simulink model "adapHCS_model"  (R2022b)
settings: Solver=VariableStepAuto  StartTime=0.0  StopTime=t_sample*n_sample  MaxStep=15  MinStep=10  RelTol=1e-3
values from neighbouring files (symbols this model uses):
  air_den = 1.225    [wind_turbine_parameters.m]
  l1 = 56    [wind_turbine_parameters.m]
  t_sample = 10*60    (= 600)    [wind_turbine_parameters.m]
undefined symbols (not defined in the file or in its folder): pitch_deg
libraries: simulink x1
settings Model: PacingRate=1000  Creator=luan  LastModifiedBy=marina
settings SolverCC: ZeroCrossAlgorithm=Adaptive
settings DebuggingCC: IgnoredZcDiagnostic=none
settings ConfigComp: CovScope=ReferencedModels

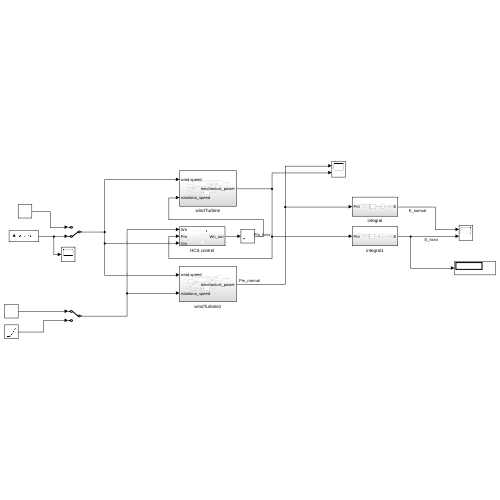
[thumbnail: Simulink's stored preview of the top-level diagram]
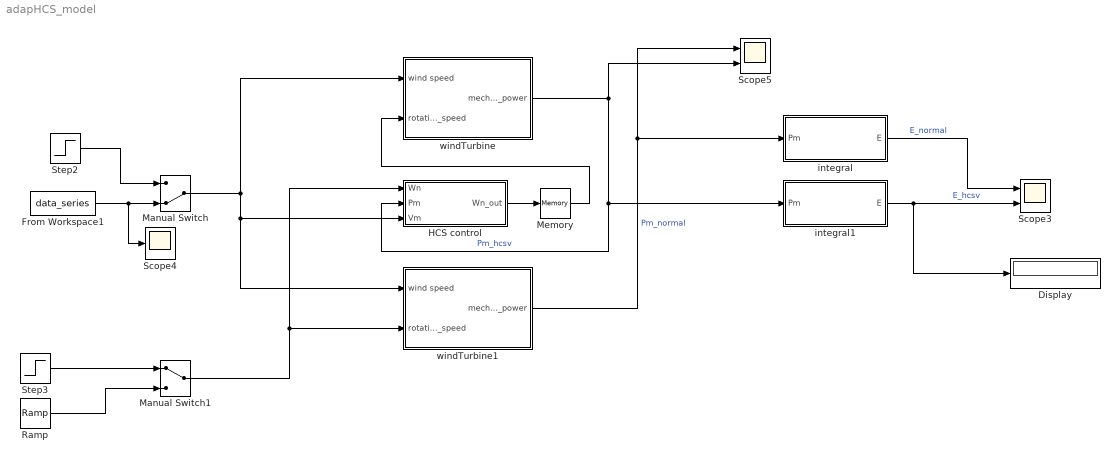
== system adapHCS_model ==
  Display : Display
  From Workspace1 : FromWorkspace  VariableName=data_series  SampleTime=t_sample  OutputAfterFinalValue=Setting to zero
  HCS control : Subsystem
  Manual Switch : ManualSwitch  CurrentSetting=0
  Manual Switch1 : ManualSwitch
  Memory : Memory
  Ramp : simulink/Sources/Ramp  slope=0.000007  start=0  InitialOutput=0.0001
  Scope3 : Scope  NumInputPorts=2
  Scope4 : Scope
  Scope5 : Scope  NumInputPorts=2
  Step2 : Step  Time=0  After=10  SampleTime=0
  Step3 : Step  Time=0  SampleTime=0
  integral : Subsystem
  integral1 : Subsystem
  windTurbine : Subsystem
  windTurbine1 : Subsystem
  wires:
  windTurbine1/1(mechanical_power) -> Scope5/1, integral/1(Pm)  "Pm_normal"
  windTurbine/1(mechanical_power) -> Scope5/2, HCS control/2(Pm), integral1/1(Pm)  "Pm_hcsv"
  Step2/1 -> Manual Switch/1
  From Workspace1/1 -> Scope4/1, Manual Switch/2
  Step3/1 -> Manual Switch1/1
  Ramp/1 -> Manual Switch1/2
  HCS control/1(Wn_out) -> Memory/1
  integral1/1(E) -> Display/1, Scope3/2  "E_hcsv"
  Memory/1 -> windTurbine/2(rotationa_speed)
  integral/1(E) -> Scope3/1  "E_normal"
  Manual Switch1/1 -> HCS control/1(Wn), windTurbine1/2(rotationa_speed)
  Manual Switch/1 -> windTurbine/1(wind speed), windTurbine1/1(wind speed), HCS control/3(Vm)

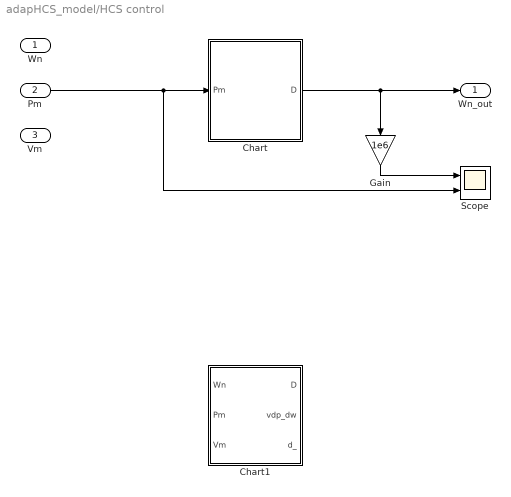
== system adapHCS_model/HCS control ==
  Wn : Inport
  Pm : Inport  Port=2
  Vm : Inport  Port=3
  Chart : Stateflow chart  TreatAsAtomicUnit=on
  Chart1 : Stateflow chart  TreatAsAtomicUnit=on
  Gain : Gain  Gain=1e6
  Scope : Scope  NumInputPorts=2
  Wn_out : Outport
  wires:
  Chart/1(D) -> Gain/1, Wn_out/1
  Pm/1 -> Scope/2, Chart/1(Pm)
  Gain/1 -> Scope/1

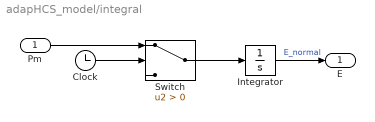
== system adapHCS_model/integral ==
  Pm : Inport
  Clock : Clock
  Integrator : Integrator
  Switch : Switch  Criteria=u2 > Threshold  SaturateOnIntegerOverflow=off  InputSameDT=off
  E : Outport
  wires:
  Switch/1 -> Integrator/1
  Clock/1 -> Switch/2
  Pm/1 -> Switch/1
  Integrator/1 -> E/1  "E_normal"

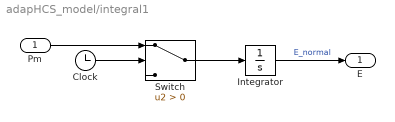
== system adapHCS_model/integral1 ==
  Pm : Inport
  Clock : Clock
  Integrator : Integrator
  Switch : Switch  Criteria=u2 > Threshold  SaturateOnIntegerOverflow=off  InputSameDT=off
  E : Outport
  wires:
  Integrator/1 -> E/1  "E_normal"
  Pm/1 -> Switch/1
  Clock/1 -> Switch/2
  Switch/1 -> Integrator/1

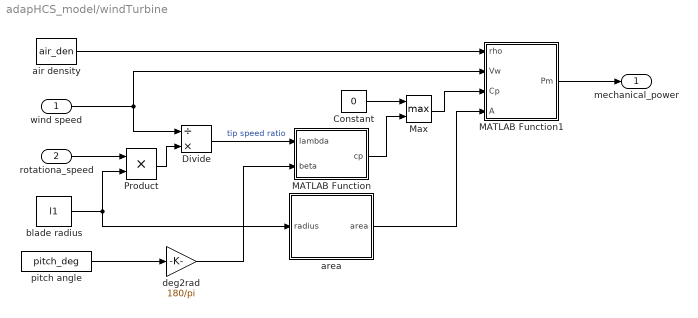
== system adapHCS_model/windTurbine ==
  wind speed : Inport
  rotationa_speed : Inport  Port=2
  Constant : Constant  Value=0
  Divide : Product  Inputs=/*
  MATLAB Function : MATLAB Function  TreatAsAtomicUnit=on
  MATLAB Function1 : MATLAB Function  TreatAsAtomicUnit=on
  Max : MinMax  Function=max  Inputs=2
  Product : Product
  air density : Constant  Value=air_den
  area : Subsystem
  blade radius : Constant  Value=l1
  deg2rad : Gain  Gain=180/pi
  pitch angle : Constant  Value=pitch_deg
  mechanical_power : Outport
  wires:
  Product/1 -> Divide/2
  wind speed/1 -> Divide/1, MATLAB Function1/2(Vw)
  Divide/1 -> MATLAB Function/1(lambda)  "tip speed ratio"
  MATLAB Function1/1(Pm) -> mechanical_power/1
  rotationa_speed/1 -> Product/1
  air density/1 -> MATLAB Function1/1(rho)
  area/1(area) -> MATLAB Function1/4(A)
  blade radius/1 -> Product/2, area/1(radius)
  deg2rad/1 -> MATLAB Function/2(beta)
  Max/1 -> MATLAB Function1/3(Cp)
  MATLAB Function/1(cp) -> Max/2
  Constant/1 -> Max/1
  pitch angle/1 -> deg2rad/1

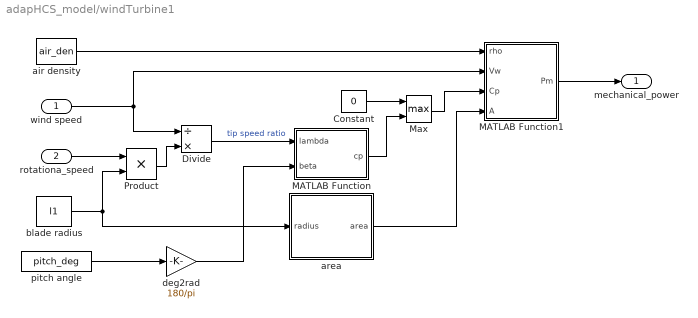
== system adapHCS_model/windTurbine1 ==
  wind speed : Inport
  rotationa_speed : Inport  Port=2
  Constant : Constant  Value=0
  Divide : Product  Inputs=/*
  MATLAB Function : MATLAB Function  TreatAsAtomicUnit=on
  MATLAB Function1 : MATLAB Function  TreatAsAtomicUnit=on
  Max : MinMax  Function=max  Inputs=2
  Product : Product
  air density : Constant  Value=air_den
  area : Subsystem
  blade radius : Constant  Value=l1
  deg2rad : Gain  Gain=180/pi
  pitch angle : Constant  Value=pitch_deg
  mechanical_power : Outport
  wires:
  Product/1 -> Divide/2
  wind speed/1 -> Divide/1, MATLAB Function1/2(Vw)
  Divide/1 -> MATLAB Function/1(lambda)  "tip speed ratio"
  MATLAB Function1/1(Pm) -> mechanical_power/1
  rotationa_speed/1 -> Product/1
  air density/1 -> MATLAB Function1/1(rho)
  area/1(area) -> MATLAB Function1/4(A)
  blade radius/1 -> Product/2, area/1(radius)
  deg2rad/1 -> MATLAB Function/2(beta)
  Max/1 -> MATLAB Function1/3(Cp)
  MATLAB Function/1(cp) -> Max/2
  Constant/1 -> Max/1
  pitch angle/1 -> deg2rad/1

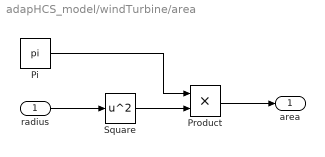
== system adapHCS_model/windTurbine/area ==
  radius : Inport
  Pi : Constant  Value=pi  OutDataTypeStr=Inherit: Inherit via back propagation
  Product : Product
  Square : Math  Operator=square
  area : Outport
  wires:
  radius/1 -> Square/1
  Square/1 -> Product/2
  Pi/1 -> Product/1
  Product/1 -> area/1

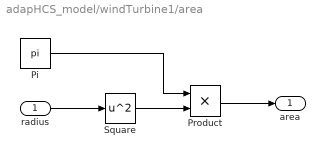
== system adapHCS_model/windTurbine1/area ==
  radius : Inport
  Pi : Constant  Value=pi  OutDataTypeStr=Inherit: Inherit via back propagation
  Product : Product
  Square : Math  Operator=square
  area : Outport
  wires:
  radius/1 -> Square/1
  Square/1 -> Product/2
  Pi/1 -> Product/1
  Product/1 -> area/1

== stateflow chart adapHCS_model/HCS control/Chart ==
  state init_
    entry:
    D = 1;
    pt_1 = Pm;
    direction = 1;
  state perturb_
    entry:
    D = D + d_;
    D = max(D, 0);
    pt_1 = Pm;
  state measure
    entry:
    dp = Pm - pt_1;
  state keep_direction
    entry:
    direction = direction;
  state update
    entry:
    d_ = direction * Gamma * abs(dp);
  state change_direction
    entry:
    direction = -1* direction;
  state perturb
    entry:
    d_ = randn(1)/500;
    direction = d_/abs(d_);
  (junction 73) -> (junction 74)
  (default) -> init_
  (junction 74) -> measure
  (junction 77) -> (junction 73)
  update -> perturb_
  init_ -> measure
  measure -> keep_direction [order 2] : [dp > Tr]
  keep_direction -> update
  perturb_ -> (junction 77) : [after(delay,sec)]
  (junction 99) -> update
  measure -> perturb [order 3]
  measure -> (junction 95) [order 1] : [dp < -Tr]
  (junction 121) -> perturb_
  (junction 95) -> change_direction
  change_direction -> (junction 99)
  perturb -> (junction 121)
  data: Pm input; D output; delay constant double =30; pt_1 local =1000; dp local; Gamma constant double =1e-7; d_ local; direction local; Tr constant double

== matlab function adapHCS_model/windTurbine/MATLAB Function ==
  data: lambda input; cp output; beta input
function cp = fcn(lambda, beta)

k = load('coefficients.mat');
lambda_i =  1/(1/(lambda + 0.08*beta) - 0.035/(1+beta*beta*beta));

% Debug
% lambda_i
% k.k1 *(k.k2/lambda_i - k.k3*beta - k.k4*power(beta, k.k5) -k.k6)*exp(-k.k7/lambda_i)

cp = k.k1 *(k.k2/lambda_i - k.k3*beta - k.k4*power(beta, k.k5) -k.k6)*exp(-k.k7/lambda_i);

== matlab function adapHCS_model/windTurbine1/MATLAB Function ==
  data: lambda input; cp output; beta input
function cp = fcn(lambda, beta)

k = load('coefficients.mat');
lambda_i =  1/(1/(lambda + 0.08*beta) - 0.035/(1+beta*beta*beta));

% Debug
% lambda_i
% k.k1 *(k.k2/lambda_i - k.k3*beta - k.k4*power(beta, k.k5) -k.k6)*exp(-k.k7/lambda_i)

cp = k.k1 *(k.k2/lambda_i - k.k3*beta - k.k4*power(beta, k.k5) -k.k6)*exp(-k.k7/lambda_i);

== matlab function adapHCS_model/windTurbine1/MATLAB Function1 ==
  data: rho input; Vw input; Pm output; Cp input; A input
function Pm = fcn(rho, Vw, Cp, A)

Pm = 0.5* Cp* rho* A* power(Vw, 3);

== matlab function adapHCS_model/windTurbine/MATLAB Function1 ==
  data: rho input; Vw input; Pm output; Cp input; A input
function Pm = fcn(rho, Vw, Cp, A)

Pm = 0.5* Cp* rho* A* power(Vw, 3);

== stateflow chart adapHCS_model/HCS control/Chart1 ==
  state stationary
    entry:
    D = Wn;
  state measure
    entry:
    dp = Pm - pt_1;
    dw = D-wn_1;
    pt_1 = Pm;
    wn_1 = D;
    vdp_dw =  Vm*dp/dw;
  state decrease
    entry:
  state decrease_a_lot
    entry:
    d_ = - d_lot;
  state init_
    entry:
    D = Wn;
    pt_1 = 0;
    wn_1 = 0;
    vdp_dw_1 = 0;
  state decrease_a_bit
    entry:
    d_ = - d_bit;
  state perturb_
    entry:
    D = D + d_;
    vdp_dw_1 = vdp_dw;
  state increase_a_bit
    entry:
    d_ = d_bit;
  state increase
    entry:
  state increase_a_lot
    entry:
    d_ = d_lot;
  measure -> stationary [order 3] : [dp==0]
  stationary -> measure : [after(delay,sec)]
  (junction 73) -> (junction 74)
  (junction 74) -> measure
  (junction 77) -> (junction 73)
  (default) -> init_
  decrease_a_lot -> (junction 66)
  measure -> decrease [order 2] : [dp < 0]
  decrease -> decrease_a_lot [order 2] : [Pm < vdp_dw_1]
  (junction 66) -> perturb_
  init_ -> measure
  decrease -> decrease_a_bit [order 1] : [Pm > vdp_dw_1]
  measure -> increase [order 1] : [dp > 0]
  decrease_a_bit -> (junction 70)
  (junction 70) -> perturb_
  perturb_ -> (junction 77) : [after(delay,sec)]
  (junction 63) -> perturb_
  (junction 60) -> perturb_
  increase_a_bit -> (junction 63)
  increase -> increase_a_bit [order 1] : [Pm > vdp_dw_1]
  increase -> (junction 45) [order 2] : [Pm < vdp_dw_1]
  (junction 45) -> increase_a_lot
  increase_a_lot -> (junction 60)
  data: Wn input; Pm input; D output; delay constant double =60; d_bit constant double =0.005; pt_1 local; wn_1 local; d_lot constant double =0.15; Vm input; dw local; vdp_dw output; d_ output; vdp_dw_1 local; dp local; Gamma constant double
